simulink model "IEEE39_IBR_FrequencyControl_Primary_2020a"  (R2020a)
settings: Solver=VariableStepAuto  StartTime=0.0  StopTime=30  RelTol=1e-3
InitFcn:
  | IEEE39data_FrencyControl_primary;
undefined symbols (not defined in the file): Fref, IBR_data, line, Sbase, t_start_disturbance, Vbase
libraries: powerlib x203, powerlib_meascontrol x81, powerlib_extras x27, simulink x14
(part 5 of 5)

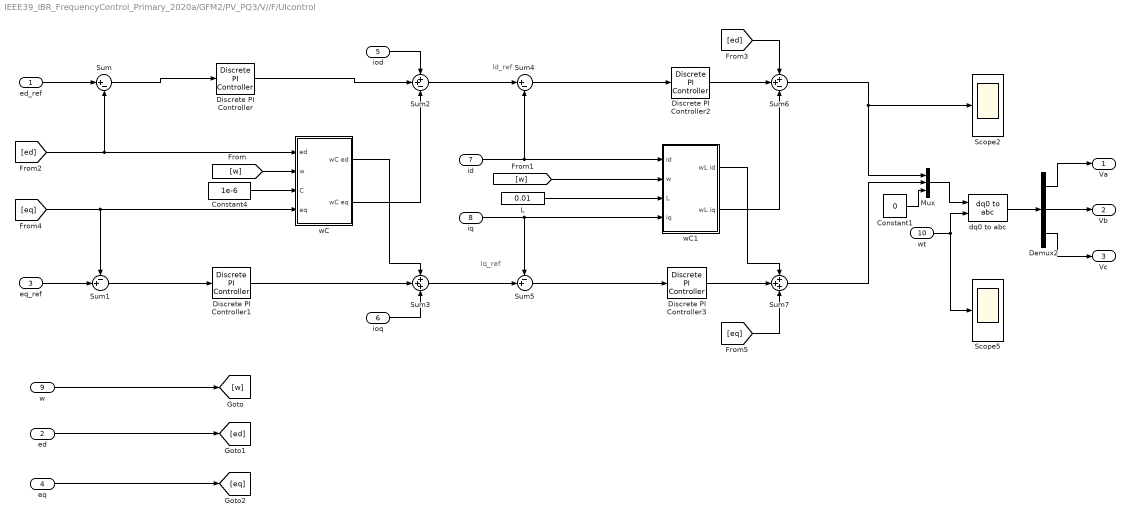
== system IEEE39_IBR_FrequencyControl_Primary_2020a/GFM2/PV_PQ3/V//F/UIcontrol ==
  note: Id_ref
  note: Iq_ref
  ed_ref : Inport
  ed : Inport  Port=2
  eq_ref : Inport  Port=3
  eq : Inport  Port=4
  iod : Inport  Port=5
  ioq : Inport  Port=6
  id : Inport  Port=7
  iq : Inport  Port=8
  w : Inport  Port=9
  "wt " : Inport  Port=10
  Constant1 : Constant  Value=0
  Constant4 : Constant  Value=1e-6
  Demux2 : Demux  Outputs=3
  Discrete PI Controller : powerlib_extras/Discrete  Control Blocks/Discrete PI Controller  Kp=0.3  Ki=0.8  Par_Limits=[1e6 -1e6]  Init=0  Ts=2e-4
  Discrete PI Controller1 : powerlib_extras/Discrete  Control Blocks/Discrete PI Controller  Kp=0.3  Ki=0.8  Par_Limits=[1e6 -1e6]  Init=0  Ts=2e-4
  Discrete PI Controller2 : powerlib_extras/Discrete  Control Blocks/Discrete PI Controller  Kp=2.5  Ki=12.5  Par_Limits=[1e6 -1e6]  Init=0  Ts=2e-4
  Discrete PI Controller3 : powerlib_extras/Discrete  Control Blocks/Discrete PI Controller  Kp=2.5  Ki=12.5  Par_Limits=[1e6 -1e6]  Init=0  Ts=2e-4
  L : Constant  Value=0.01
  Mux : Mux  Inputs=3
  Scope2 : Scope
  Scope5 : Scope
  Sum : Sum  Inputs=|+-
  Sum1 : Sum  Inputs=-+|
  Sum2 : Sum  Inputs=++-
  Sum3 : Sum  Inputs=+++
  Sum4 : Sum  Inputs=|+-
  Sum5 : Sum  Inputs=-+|
  Sum6 : Sum  Inputs=++-
  Sum7 : Sum  Inputs=+++
  dq0 to abc : powerlib_meascontrol/Transformations/dq0 to abc  Alignment=90 degrees behind phase A axis
  wC : Subsystem
  wC1 : Subsystem
  Va : Outport
  Vb : Outport  Port=2
  Vc : Outport  Port=3
  wires:
  [ed] -> wC/1(ed), Sum/2
  Mux/1 -> dq0 to abc/1
  Demux2/1 -> Va/1
  Demux2/2 -> Vb/1
  Demux2/3 -> Vc/1
  dq0 to abc/1 -> Demux2/1
  Constant4/1 -> wC/3(C)
  [w] -> wC/2(w)
  [eq] -> wC/4(eq), Sum1/1
  eq_ref/1 -> Sum1/2
  Sum2/1 -> Sum4/1
  L/1 -> wC1/3(L)
  Discrete PI Controller3/1 -> Sum7/2
  Discrete PI Controller2/1 -> Sum6/2
  w/1 -> [w]
  [w] -> wC1/2(w)
  ed/1 -> [ed]
  eq/1 -> [eq]
  Sum6/1 -> Scope2/1, Mux/1
  Sum7/1 -> Mux/2
  Sum3/1 -> Sum5/2
  Constant1/1 -> Mux/3
  iq/1 -> Sum5/1, wC1/4(iq)
  [eq] -> Sum7/3
  [ed] -> Sum6/1
  id/1 -> wC1/1(id), Sum4/2
  wC/1(wC ed) -> Sum3/1
  ioq/1 -> Sum3/3
  iod/1 -> Sum2/1
  wC/2(wC eq) -> Sum2/3
  wC1/1(wL id) -> Sum7/1
  wC1/2(wL iq) -> Sum6/3
  Sum/1 -> Discrete PI Controller/1
  Discrete PI Controller/1 -> Sum2/2
  Sum1/1 -> Discrete PI Controller1/1
  Discrete PI Controller1/1 -> Sum3/2
  Sum4/1 -> Discrete PI Controller2/1
  Sum5/1 -> Discrete PI Controller3/1
  ed_ref/1 -> Sum/1
  "wt "/1 -> Scope5/1, dq0 to abc/2

== system IEEE39_IBR_FrequencyControl_Primary_2020a/GFM3/PV_PQ3/V//F/Subsystem ==
  note: w
  eo : Inport
  io : Inport  Port=2
  i : Inport  Port=3
  f : Inport  Port=4
  Init_Phase_degree : Inport  Port=5
  Add : Sum
  Demux : Demux  Outputs=3
  Demux1 : Demux  Outputs=3
  Demux2 : Demux  Outputs=3
  Gain1 : Gain  Gain=2*pi
  Gain2 : Gain  Gain=pi/180
  Integrator : Integrator
  Scope2 : Scope
  Terminator1 : Terminator
  Terminator2 : Terminator
  Terminator3 : Terminator
  abc to dq0 : powerlib_meascontrol/Transformations/abc to dq0  Alignment=90 degrees behind phase A axis
  abc to dq1 : powerlib_meascontrol/Transformations/abc to dq0  Alignment=90 degrees behind phase A axis
  abc to dq2 : powerlib_meascontrol/Transformations/abc to dq0  Alignment=90 degrees behind phase A axis
  eod : Outport  VectorParamsAs1DForOutWhenUnconnected=off
  eoq : Outport  Port=2  VectorParamsAs1DForOutWhenUnconnected=off
  iod : Outport  Port=3  VectorParamsAs1DForOutWhenUnconnected=off
  ioq : Outport  Port=4  VectorParamsAs1DForOutWhenUnconnected=off
  id : Outport  Port=5  VectorParamsAs1DForOutWhenUnconnected=off
  iq : Outport  Port=6  VectorParamsAs1DForOutWhenUnconnected=off
  w : Outport  Port=7  VectorParamsAs1DForOutWhenUnconnected=off
  "wt " : Outport  Port=8  VectorParamsAs1DForOutWhenUnconnected=off
  wires:
  eo/1 -> abc to dq0/1
  i/1 -> abc to dq1/1
  f/1 -> Gain1/1
  Add/1 -> "wt "/1, abc to dq1/2, abc to dq2/2, abc to dq0/2
  Demux1/1 -> id/1
  Demux1/2 -> iq/1
  Demux1/3 -> Terminator3/1
  Demux/1 -> eod/1
  Demux/2 -> eoq/1
  Demux/3 -> Terminator1/1
  io/1 -> abc to dq2/1
  Demux2/3 -> Terminator2/1
  Gain1/1 -> Integrator/1, w/1
  Demux2/1 -> iod/1
  Demux2/2 -> ioq/1
  abc to dq2/1 -> Demux2/1
  abc to dq1/1 -> Demux1/1
  abc to dq0/1 -> Demux/1
  Integrator/1 -> Add/1
  Init_Phase_degree/1 -> Gain2/1
  Gain2/1 -> Add/2, Scope2/1

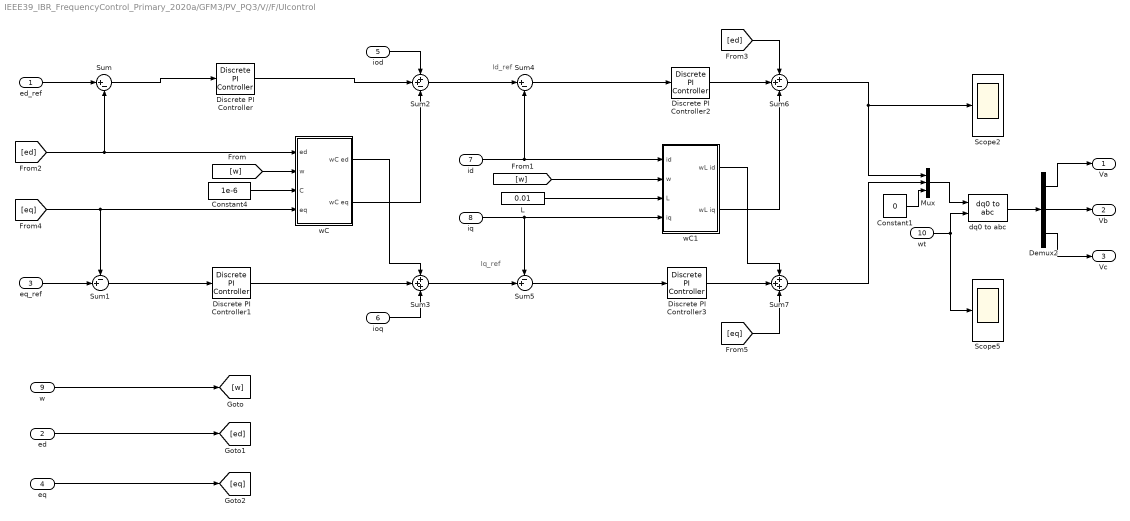
== system IEEE39_IBR_FrequencyControl_Primary_2020a/GFM3/PV_PQ3/V//F/UIcontrol ==
  note: Id_ref
  note: Iq_ref
  ed_ref : Inport
  ed : Inport  Port=2
  eq_ref : Inport  Port=3
  eq : Inport  Port=4
  iod : Inport  Port=5
  ioq : Inport  Port=6
  id : Inport  Port=7
  iq : Inport  Port=8
  w : Inport  Port=9
  "wt " : Inport  Port=10
  Constant1 : Constant  Value=0
  Constant4 : Constant  Value=1e-6
  Demux2 : Demux  Outputs=3
  Discrete PI Controller : powerlib_extras/Discrete  Control Blocks/Discrete PI Controller  Kp=0.3  Ki=0.8  Par_Limits=[1e6 -1e6]  Init=0  Ts=2e-4
  Discrete PI Controller1 : powerlib_extras/Discrete  Control Blocks/Discrete PI Controller  Kp=0.3  Ki=0.8  Par_Limits=[1e6 -1e6]  Init=0  Ts=2e-4
  Discrete PI Controller2 : powerlib_extras/Discrete  Control Blocks/Discrete PI Controller  Kp=2.5  Ki=12.5  Par_Limits=[1e6 -1e6]  Init=0  Ts=2e-4
  Discrete PI Controller3 : powerlib_extras/Discrete  Control Blocks/Discrete PI Controller  Kp=2.5  Ki=12.5  Par_Limits=[1e6 -1e6]  Init=0  Ts=2e-4
  L : Constant  Value=0.01
  Mux : Mux  Inputs=3
  Scope2 : Scope
  Scope5 : Scope
  Sum : Sum  Inputs=|+-
  Sum1 : Sum  Inputs=-+|
  Sum2 : Sum  Inputs=++-
  Sum3 : Sum  Inputs=+++
  Sum4 : Sum  Inputs=|+-
  Sum5 : Sum  Inputs=-+|
  Sum6 : Sum  Inputs=++-
  Sum7 : Sum  Inputs=+++
  dq0 to abc : powerlib_meascontrol/Transformations/dq0 to abc  Alignment=90 degrees behind phase A axis
  wC : Subsystem
  wC1 : Subsystem
  Va : Outport
  Vb : Outport  Port=2
  Vc : Outport  Port=3
  wires:
  [ed] -> wC/1(ed), Sum/2
  Mux/1 -> dq0 to abc/1
  Demux2/1 -> Va/1
  Demux2/2 -> Vb/1
  Demux2/3 -> Vc/1
  dq0 to abc/1 -> Demux2/1
  Constant4/1 -> wC/3(C)
  [w] -> wC/2(w)
  [eq] -> wC/4(eq), Sum1/1
  eq_ref/1 -> Sum1/2
  Sum2/1 -> Sum4/1
  L/1 -> wC1/3(L)
  Discrete PI Controller3/1 -> Sum7/2
  Discrete PI Controller2/1 -> Sum6/2
  w/1 -> [w]
  [w] -> wC1/2(w)
  ed/1 -> [ed]
  eq/1 -> [eq]
  Sum6/1 -> Scope2/1, Mux/1
  Sum7/1 -> Mux/2
  Sum3/1 -> Sum5/2
  Constant1/1 -> Mux/3
  iq/1 -> Sum5/1, wC1/4(iq)
  [eq] -> Sum7/3
  [ed] -> Sum6/1
  id/1 -> wC1/1(id), Sum4/2
  wC/1(wC ed) -> Sum3/1
  ioq/1 -> Sum3/3
  iod/1 -> Sum2/1
  wC/2(wC eq) -> Sum2/3
  wC1/1(wL id) -> Sum7/1
  wC1/2(wL iq) -> Sum6/3
  Sum/1 -> Discrete PI Controller/1
  Discrete PI Controller/1 -> Sum2/2
  Sum1/1 -> Discrete PI Controller1/1
  Discrete PI Controller1/1 -> Sum3/2
  Sum4/1 -> Discrete PI Controller2/1
  Sum5/1 -> Discrete PI Controller3/1
  ed_ref/1 -> Sum/1
  "wt "/1 -> Scope5/1, dq0 to abc/2

== system IEEE39_IBR_FrequencyControl_Primary_2020a/GFM4/PV_PQ3/V//F/Subsystem ==
  note: w
  eo : Inport
  io : Inport  Port=2
  i : Inport  Port=3
  f : Inport  Port=4
  Init_Phase_degree : Inport  Port=5
  Add : Sum
  Demux : Demux  Outputs=3
  Demux1 : Demux  Outputs=3
  Demux2 : Demux  Outputs=3
  Gain1 : Gain  Gain=2*pi
  Gain2 : Gain  Gain=pi/180
  Integrator : Integrator
  Scope2 : Scope
  Terminator1 : Terminator
  Terminator2 : Terminator
  Terminator3 : Terminator
  abc to dq0 : powerlib_meascontrol/Transformations/abc to dq0  Alignment=90 degrees behind phase A axis
  abc to dq1 : powerlib_meascontrol/Transformations/abc to dq0  Alignment=90 degrees behind phase A axis
  abc to dq2 : powerlib_meascontrol/Transformations/abc to dq0  Alignment=90 degrees behind phase A axis
  eod : Outport  VectorParamsAs1DForOutWhenUnconnected=off
  eoq : Outport  Port=2  VectorParamsAs1DForOutWhenUnconnected=off
  iod : Outport  Port=3  VectorParamsAs1DForOutWhenUnconnected=off
  ioq : Outport  Port=4  VectorParamsAs1DForOutWhenUnconnected=off
  id : Outport  Port=5  VectorParamsAs1DForOutWhenUnconnected=off
  iq : Outport  Port=6  VectorParamsAs1DForOutWhenUnconnected=off
  w : Outport  Port=7  VectorParamsAs1DForOutWhenUnconnected=off
  "wt " : Outport  Port=8  VectorParamsAs1DForOutWhenUnconnected=off
  wires:
  eo/1 -> abc to dq0/1
  i/1 -> abc to dq1/1
  f/1 -> Gain1/1
  Add/1 -> "wt "/1, abc to dq1/2, abc to dq2/2, abc to dq0/2
  Demux1/1 -> id/1
  Demux1/2 -> iq/1
  Demux1/3 -> Terminator3/1
  Demux/1 -> eod/1
  Demux/2 -> eoq/1
  Demux/3 -> Terminator1/1
  io/1 -> abc to dq2/1
  Demux2/3 -> Terminator2/1
  Gain1/1 -> Integrator/1, w/1
  Demux2/1 -> iod/1
  Demux2/2 -> ioq/1
  abc to dq2/1 -> Demux2/1
  abc to dq1/1 -> Demux1/1
  abc to dq0/1 -> Demux/1
  Integrator/1 -> Add/1
  Init_Phase_degree/1 -> Gain2/1
  Gain2/1 -> Add/2, Scope2/1

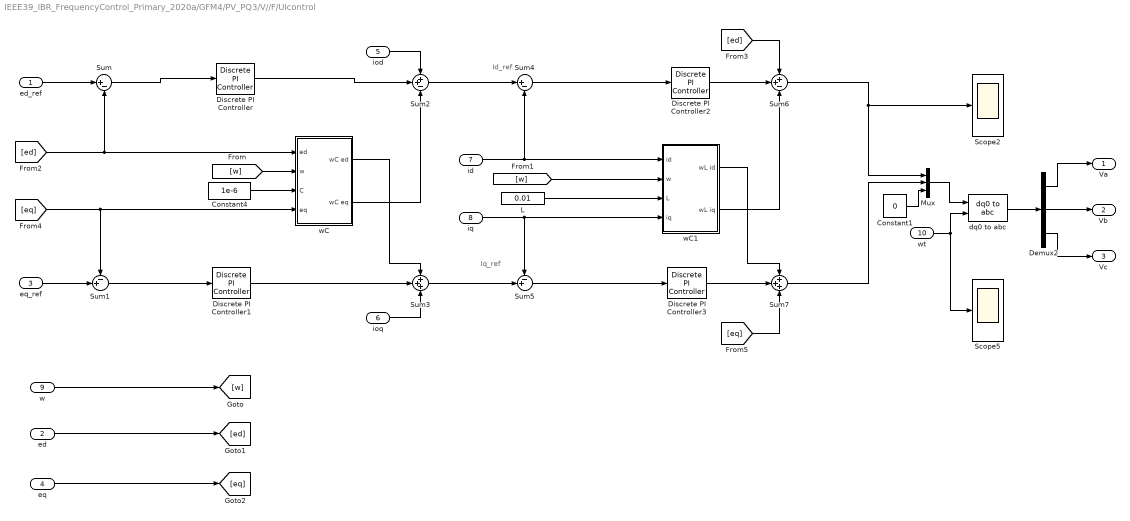
== system IEEE39_IBR_FrequencyControl_Primary_2020a/GFM4/PV_PQ3/V//F/UIcontrol ==
  note: Id_ref
  note: Iq_ref
  ed_ref : Inport
  ed : Inport  Port=2
  eq_ref : Inport  Port=3
  eq : Inport  Port=4
  iod : Inport  Port=5
  ioq : Inport  Port=6
  id : Inport  Port=7
  iq : Inport  Port=8
  w : Inport  Port=9
  "wt " : Inport  Port=10
  Constant1 : Constant  Value=0
  Constant4 : Constant  Value=1e-6
  Demux2 : Demux  Outputs=3
  Discrete PI Controller : powerlib_extras/Discrete  Control Blocks/Discrete PI Controller  Kp=0.3  Ki=0.8  Par_Limits=[1e6 -1e6]  Init=0  Ts=2e-4
  Discrete PI Controller1 : powerlib_extras/Discrete  Control Blocks/Discrete PI Controller  Kp=0.3  Ki=0.8  Par_Limits=[1e6 -1e6]  Init=0  Ts=2e-4
  Discrete PI Controller2 : powerlib_extras/Discrete  Control Blocks/Discrete PI Controller  Kp=2.5  Ki=12.5  Par_Limits=[1e6 -1e6]  Init=0  Ts=2e-4
  Discrete PI Controller3 : powerlib_extras/Discrete  Control Blocks/Discrete PI Controller  Kp=2.5  Ki=12.5  Par_Limits=[1e6 -1e6]  Init=0  Ts=2e-4
  L : Constant  Value=0.01
  Mux : Mux  Inputs=3
  Scope2 : Scope
  Scope5 : Scope
  Sum : Sum  Inputs=|+-
  Sum1 : Sum  Inputs=-+|
  Sum2 : Sum  Inputs=++-
  Sum3 : Sum  Inputs=+++
  Sum4 : Sum  Inputs=|+-
  Sum5 : Sum  Inputs=-+|
  Sum6 : Sum  Inputs=++-
  Sum7 : Sum  Inputs=+++
  dq0 to abc : powerlib_meascontrol/Transformations/dq0 to abc  Alignment=90 degrees behind phase A axis
  wC : Subsystem
  wC1 : Subsystem
  Va : Outport
  Vb : Outport  Port=2
  Vc : Outport  Port=3
  wires:
  [ed] -> wC/1(ed), Sum/2
  Mux/1 -> dq0 to abc/1
  Demux2/1 -> Va/1
  Demux2/2 -> Vb/1
  Demux2/3 -> Vc/1
  dq0 to abc/1 -> Demux2/1
  Constant4/1 -> wC/3(C)
  [w] -> wC/2(w)
  [eq] -> wC/4(eq), Sum1/1
  eq_ref/1 -> Sum1/2
  Sum2/1 -> Sum4/1
  L/1 -> wC1/3(L)
  Discrete PI Controller3/1 -> Sum7/2
  Discrete PI Controller2/1 -> Sum6/2
  w/1 -> [w]
  [w] -> wC1/2(w)
  ed/1 -> [ed]
  eq/1 -> [eq]
  Sum6/1 -> Scope2/1, Mux/1
  Sum7/1 -> Mux/2
  Sum3/1 -> Sum5/2
  Constant1/1 -> Mux/3
  iq/1 -> Sum5/1, wC1/4(iq)
  [eq] -> Sum7/3
  [ed] -> Sum6/1
  id/1 -> wC1/1(id), Sum4/2
  wC/1(wC ed) -> Sum3/1
  ioq/1 -> Sum3/3
  iod/1 -> Sum2/1
  wC/2(wC eq) -> Sum2/3
  wC1/1(wL id) -> Sum7/1
  wC1/2(wL iq) -> Sum6/3
  Sum/1 -> Discrete PI Controller/1
  Discrete PI Controller/1 -> Sum2/2
  Sum1/1 -> Discrete PI Controller1/1
  Discrete PI Controller1/1 -> Sum3/2
  Sum4/1 -> Discrete PI Controller2/1
  Sum5/1 -> Discrete PI Controller3/1
  ed_ref/1 -> Sum/1
  "wt "/1 -> Scope5/1, dq0 to abc/2

== system IEEE39_IBR_FrequencyControl_Primary_2020a/PV/PV_PQ3/Subsystem2/Subsystem1 ==
  P_ref : Inport
  Q_ref : Inport  Port=2
  Ud : Inport  Port=3
  Divide5 : Product  Inputs=*/
  Divide6 : Product  Inputs=*/
  Gain1 : Gain  Gain=-2/3
  Gain2 : Gain  Gain=2/3
  Id_ref : Outport  VectorParamsAs1DForOutWhenUnconnected=off
  Iq_ref : Outport  Port=2  VectorParamsAs1DForOutWhenUnconnected=off
  wires:
  Q_ref/1 -> Divide6/1
  Divide6/1 -> Gain1/1
  P_ref/1 -> Divide5/1
  Gain1/1 -> Iq_ref/1
  Divide5/1 -> Gain2/1
  Gain2/1 -> Id_ref/1
  Ud/1 -> Divide6/2, Divide5/2

== system IEEE39_IBR_FrequencyControl_Primary_2020a/PV/PV_PQ3/Subsystem2/WL ==
  In1 : Inport
  freq : Inport  Port=2
  L : Inport  Port=3
  2pai : Constant  Value=2*pi
  Product : Product  Inputs=**
  Product1 : Product  Inputs=***
  Out1 : Outport  VectorParamsAs1DForOutWhenUnconnected=off
  wires:
  2pai/1 -> Product/2
  L/1 -> Product1/3
  freq/1 -> Product/1
  Product1/1 -> Out1/1
  Product/1 -> Product1/2
  In1/1 -> Product1/1

== system IEEE39_IBR_FrequencyControl_Primary_2020a/PV/PV_PQ3/Subsystem2/WL1 ==
  In1 : Inport
  freq : Inport  Port=2
  L : Inport  Port=3
  2pai : Constant  Value=2*pi
  Product : Product
  Product1 : Product  Inputs=3
  Out1 : Outport  VectorParamsAs1DForOutWhenUnconnected=off
  wires:
  2pai/1 -> Product/2
  L/1 -> Product1/3
  freq/1 -> Product/1
  Product1/1 -> Out1/1
  Product/1 -> Product1/2
  In1/1 -> Product1/1

== system IEEE39_IBR_FrequencyControl_Primary_2020a/GFM1/PV_PQ3/V//F/UIcontrol/wC ==
  ed : Inport
  w : Inport  Port=2
  C : Inport  Port=3
  eq : Inport  Port=4
  Product1 : Product  Inputs=3
  Product2 : Product  Inputs=3
  wC ed : Outport  VectorParamsAs1DForOutWhenUnconnected=off
  wC eq : Outport  Port=2  VectorParamsAs1DForOutWhenUnconnected=off
  wires:
  C/1 -> Product1/3, Product2/2
  Product1/1 -> wC ed/1
  w/1 -> Product1/2, Product2/1
  ed/1 -> Product1/1
  eq/1 -> Product2/3
  Product2/1 -> wC eq/1

== system IEEE39_IBR_FrequencyControl_Primary_2020a/GFM1/PV_PQ3/V//F/UIcontrol/wC1 ==
  id : Inport
  w : Inport  Port=2
  L : Inport  Port=3
  iq : Inport  Port=4
  Product1 : Product  Inputs=***
  Product2 : Product  Inputs=***
  wL id : Outport  VectorParamsAs1DForOutWhenUnconnected=off
  wL iq : Outport  Port=2  VectorParamsAs1DForOutWhenUnconnected=off
  wires:
  L/1 -> Product1/3, Product2/2
  Product1/1 -> wL id/1
  w/1 -> Product1/2, Product2/1
  id/1 -> Product1/1
  iq/1 -> Product2/3
  Product2/1 -> wL iq/1

== system IEEE39_IBR_FrequencyControl_Primary_2020a/GFM2/PV_PQ3/V//F/UIcontrol/wC ==
  ed : Inport
  w : Inport  Port=2
  C : Inport  Port=3
  eq : Inport  Port=4
  Product1 : Product  Inputs=3
  Product2 : Product  Inputs=3
  wC ed : Outport  VectorParamsAs1DForOutWhenUnconnected=off
  wC eq : Outport  Port=2  VectorParamsAs1DForOutWhenUnconnected=off
  wires:
  C/1 -> Product1/3, Product2/2
  Product1/1 -> wC ed/1
  w/1 -> Product1/2, Product2/1
  ed/1 -> Product1/1
  eq/1 -> Product2/3
  Product2/1 -> wC eq/1

== system IEEE39_IBR_FrequencyControl_Primary_2020a/GFM2/PV_PQ3/V//F/UIcontrol/wC1 ==
  id : Inport
  w : Inport  Port=2
  L : Inport  Port=3
  iq : Inport  Port=4
  Product1 : Product  Inputs=***
  Product2 : Product  Inputs=***
  wL id : Outport  VectorParamsAs1DForOutWhenUnconnected=off
  wL iq : Outport  Port=2  VectorParamsAs1DForOutWhenUnconnected=off
  wires:
  L/1 -> Product1/3, Product2/2
  Product1/1 -> wL id/1
  w/1 -> Product1/2, Product2/1
  id/1 -> Product1/1
  iq/1 -> Product2/3
  Product2/1 -> wL iq/1

== system IEEE39_IBR_FrequencyControl_Primary_2020a/GFM3/PV_PQ3/V//F/UIcontrol/wC ==
  ed : Inport
  w : Inport  Port=2
  C : Inport  Port=3
  eq : Inport  Port=4
  Product1 : Product  Inputs=3
  Product2 : Product  Inputs=3
  wC ed : Outport  VectorParamsAs1DForOutWhenUnconnected=off
  wC eq : Outport  Port=2  VectorParamsAs1DForOutWhenUnconnected=off
  wires:
  C/1 -> Product1/3, Product2/2
  Product1/1 -> wC ed/1
  w/1 -> Product1/2, Product2/1
  ed/1 -> Product1/1
  eq/1 -> Product2/3
  Product2/1 -> wC eq/1

== system IEEE39_IBR_FrequencyControl_Primary_2020a/GFM3/PV_PQ3/V//F/UIcontrol/wC1 ==
  id : Inport
  w : Inport  Port=2
  L : Inport  Port=3
  iq : Inport  Port=4
  Product1 : Product  Inputs=***
  Product2 : Product  Inputs=***
  wL id : Outport  VectorParamsAs1DForOutWhenUnconnected=off
  wL iq : Outport  Port=2  VectorParamsAs1DForOutWhenUnconnected=off
  wires:
  L/1 -> Product1/3, Product2/2
  Product1/1 -> wL id/1
  w/1 -> Product1/2, Product2/1
  id/1 -> Product1/1
  iq/1 -> Product2/3
  Product2/1 -> wL iq/1

== system IEEE39_IBR_FrequencyControl_Primary_2020a/GFM4/PV_PQ3/V//F/UIcontrol/wC ==
  ed : Inport
  w : Inport  Port=2
  C : Inport  Port=3
  eq : Inport  Port=4
  Product1 : Product  Inputs=3
  Product2 : Product  Inputs=3
  wC ed : Outport  VectorParamsAs1DForOutWhenUnconnected=off
  wC eq : Outport  Port=2  VectorParamsAs1DForOutWhenUnconnected=off
  wires:
  C/1 -> Product1/3, Product2/2
  Product1/1 -> wC ed/1
  w/1 -> Product1/2, Product2/1
  ed/1 -> Product1/1
  eq/1 -> Product2/3
  Product2/1 -> wC eq/1

== system IEEE39_IBR_FrequencyControl_Primary_2020a/GFM4/PV_PQ3/V//F/UIcontrol/wC1 ==
  id : Inport
  w : Inport  Port=2
  L : Inport  Port=3
  iq : Inport  Port=4
  Product1 : Product  Inputs=***
  Product2 : Product  Inputs=***
  wL id : Outport  VectorParamsAs1DForOutWhenUnconnected=off
  wL iq : Outport  Port=2  VectorParamsAs1DForOutWhenUnconnected=off
  wires:
  L/1 -> Product1/3, Product2/2
  Product1/1 -> wL id/1
  w/1 -> Product1/2, Product2/1
  id/1 -> Product1/1
  iq/1 -> Product2/3
  Product2/1 -> wL iq/1
